simulink model "nms3D_2021"  (R2021a)
settings: Solver=ode15s  StartTime=0.0  StopTime=2  MaxStep=1e-2  RelTol=1e-2
StartFcn:
  | tic
StopFcn:
  | toc
  | 
  | 
  | %if GimbalLockFlag
  |  % fprintf(2, 'Almost reached Gimbal Lock of IMU. Simulation stopped.\n')
  | %end
  | 
  | %fprintf('Elapsed time: %4.2f sec (%4.2f%% realtime)\n', a, tout(end)/a*100)
values from neighbouring files (symbols this model uses):
  Balance02 = pMod(24:29)    [AssignSimulinkParams.m]    (also in assign_parameters.m = param(26:29))
  Balance13 = pMod(30:35)    [AssignSimulinkParams.m]    (also in assign_parameters.m = param(30:33))
  BalanceTrunk = pMod(22:23)    [AssignSimulinkParams.m]    (also in assign_parameters.m = param(22:23))
  BalanceTrunkLat = param(24:25)    [assign_parameters.m]
  BalanceTrunkLatOld = pMod(43:46)    [AssignSimulinkParams.m]    (also in assign_parameters.m = param(43:46))
  BalanceTrunkOld = param(49:53)    [assign_parameters.m]
  BasisStim = pMod(1:11)    [AssignSimulinkParams.m]    (also in assign_parameters.m = param(1:11))
  CompliantLeg = pMod(12:14)    [AssignSimulinkParams.m]    (also in assign_parameters.m = param(12:14))
  CompliantLegLat = pMod(15)    [AssignSimulinkParams.m]    (also in assign_parameters.m = param(15))
  PreventKneeOverextension = pMod(16:21)    [AssignSimulinkParams.m]    (also in assign_parameters.m = param(16:21))
  SwingCompLatOld = param(47:48)    [assign_parameters.m]
  Target02 = pMod(36:38)    [AssignSimulinkParams.m]    (also in assign_parameters.m = param(34:36))
  Target02_va = pMod(49:54)    [AssignSimulinkParams.m]    (also in assign_parameters.m = param(60:65))
  Target13 = pMod(39:41)    [AssignSimulinkParams.m]    (also in assign_parameters.m = param(37:39))
  Target13_va = pMod(55:60)    [AssignSimulinkParams.m]    (also in assign_parameters.m = param(66:71))
  theta0_world = param(59)    [assign_parameters.m]
  WramameiSL_1000 = readmatrix('WSL_1000_Norm_Sigmoid_MSE_cont.csv')    [nms3D_prep.m]
  ZramameiSL_1000 = readmatrix('ZSL_1000_Norm_Sigmoid_MSE_cont.csv')    [nms3D_prep.m]
undefined symbols (not defined in the file or in its folder): ICs, mParams, X, Y, Z
libraries: nesl_utility x106, sm_lib x87, simulink x70, eeGeneralControl x28, robotmaniplib x14, dspinverses x10, robotcorelib x5, dspmathops x3, vrlib x1, pid_lib x1
(part 5 of 8)

== system nms3D_2021/CMA Data/Step Counter/count steps2 ==
  nStep-1 : Inport  LatchByDelayingOutsideSignal=on
  Trigger : TriggerPort  VariantControl=(inherit)  ZeroCross=off
  Constant : Constant
  Sum : Sum  Inputs=|++
  nStep : Outport  InitialOutput=0  VectorParamsAs1DForOutWhenUnconnected=off
  wires:
  Constant/1 -> Sum/2
  nStep-1/1 -> Sum/1
  Sum/1 -> nStep/1

== system nms3D_2021/CMA Data/check steady state/even ==
  In1 : Inport
  Trigger : TriggerPort  TriggerType=falling  VariantControl=(inherit)  ZeroCross=off
  Out1 : Outport  VectorParamsAs1DForOutWhenUnconnected=off
  wires:
  In1/1 -> Out1/1

== system nms3D_2021/CMA Data/check steady state/odd ==
  In1 : Inport
  Trigger : TriggerPort  VariantControl=(inherit)  ZeroCross=off
  Out1 : Outport  VectorParamsAs1DForOutWhenUnconnected=off
  wires:
  In1/1 -> Out1/1

== system nms3D_2021/Muscle Actuation Layer/Muscles Left/Muscle Dynamics (Vectorized)1 ==
  note: Excitation Contraction Coupling
  note: VECTORIZED Muscle-Tendon Dynamics
  lmtc [m] : Inport
  STIM : Inport  Port=2
  1 : Product  Inputs=**  InputSameDT=on  SaturateOnIntegerOverflow=on  OutDataTypeStr=Inherit: Same as first input
  1./lopt : Gain  Gain=1./mParams.muscles.loptVec  SaturateOnIntegerOverflow=on  OutDataTypeStr=Inherit: Same as input  ParamDataTypeStr=Inherit: Same as input
  1./lopt2 : Gain  Gain=1/mParams.muscles.tauA  SaturateOnIntegerOverflow=on  OutDataTypeStr=Inherit: Same as input  ParamDataTypeStr=Inherit: Same as input
  1/lslack : Gain  Gain=1./mParams.muscles.lslackVec  SaturateOnIntegerOverflow=on  OutDataTypeStr=Inherit: Same as input  ParamDataTypeStr=Inherit: Same as input
  BE force-length relation : Subsystem
  CE force-length relation : Subsystem
  CE inverse force-velocity relation : Subsystem
  Constant : Constant  Value=mParams.muscles.lslackVec
  Fmax : Gain  Gain=mParams.muscles.FmaxVec  SaturateOnIntegerOverflow=on  OutDataTypeStr=Inherit: Same as input  ParamDataTypeStr=Inherit: Same as input
  Fv = Fse / (A*Fce) : Product  Inputs=*/  InputSameDT=on  SaturateOnIntegerOverflow=on  OutDataTypeStr=Inherit: Same as first input
  Integrator : Integrator  InitialConditionSource=external  LowerSaturationLimit=0.05
  Integrator1 : Integrator  InitialConditionSource=external  LowerSaturationLimit=0.05
  PE force-length relation : Subsystem
  SE force-length relation : Subsystem
  Sum : Sum  Inputs=|+-  InputSameDT=on  SaturateOnIntegerOverflow=on  OutDataTypeStr=Inherit: Same as first input
  Sum1 : Sum  Inputs=|+-  InputSameDT=on  SaturateOnIntegerOverflow=on  OutDataTypeStr=Inherit: Same as first input
  Sum2 : Sum  Inputs=|-+  InputSameDT=on  SaturateOnIntegerOverflow=on  OutDataTypeStr=Inherit: Same as first input
  Sum3 : Sum  Inputs=+++  InputSameDT=on  SaturateOnIntegerOverflow=on  OutDataTypeStr=Inherit: Same as first input
  Sum4 : Sum  InputSameDT=on  SaturateOnIntegerOverflow=on  OutDataTypeStr=Inherit: Same as first input
  avoid div by 0 : Constant  Value=eps
  preA : Constant  Value=mParams.muscles.preA
  vmax*lopt : Gain  Gain=mParams.muscles.vmaxVec  SaturateOnIntegerOverflow=on  OutDataTypeStr=Inherit: Same as input  ParamDataTypeStr=Inherit: Same as input
  Fmtc : Outport  InitialOutput=0  VectorParamsAs1DForOutWhenUnconnected=off
  Lce : Outport  Port=2  InitialOutput=0  VectorParamsAs1DForOutWhenUnconnected=off
  Vce : Outport  Port=3  InitialOutput=0  VectorParamsAs1DForOutWhenUnconnected=off
  A : Outport  Port=4  InitialOutput=0  VectorParamsAs1DForOutWhenUnconnected=off
  ForceLengthFactor : Outport  Port=5  VectorParamsAs1DForOutWhenUnconnected=off
  tag scope: fl_L=global, fv_L=global
  wires:
  1./lopt2/1 -> Integrator1/1
  Sum1/1 -> 1./lopt2/1
  CE inverse force-velocity relation/1(v[vmax]) -> vmax*lopt/1
  Fv = Fse / (A*Fce)/1 -> CE inverse force-velocity relation/1(Fv[Fmax]), [fv_L]  "fv"
  Sum3/1 -> Fv = Fse / (A*Fce)/2
  Sum4/1 -> Fv = Fse / (A*Fce)/1
  SE force-length relation/1(fse [Fmax]) -> Fmax/1, Sum4/1
  Integrator1/1 -> Sum1/2, A/1, 1/2
  Fmax/1 -> Fmtc/1  "Fmtc"
  lmtc [m]/1 -> Sum/1, Sum2/2  "lmtc"
  vmax*lopt/1 -> Integrator/1, Vce/1  "vce"
  1./lopt/1 -> CE force-length relation/1(lce [lopt]), BE force-length relation/1(lce [lopt]), PE force-length relation/1(lce [lopt])
  Integrator/1 -> 1./lopt/1, Sum/2, Lce/1  "lce"
  1/1 -> Sum3/3
  1/lslack/1 -> SE force-length relation/1(lse [lslack])
  STIM/1 -> Sum1/1
  Sum/1 -> 1/lslack/1  "lse"
  Constant/1 -> Sum2/1
  PE force-length relation/1(fpe [Fmax]) -> Sum3/1
  BE force-length relation/1(fbe [Fmax]) -> Sum4/2
  avoid div by 0/1 -> Sum3/2
  preA/1 -> Integrator1/2
  Sum2/1 -> Integrator/2
  CE force-length relation/1(fce [Fmax]) -> [fl_L], ForceLengthFactor/1, 1/1

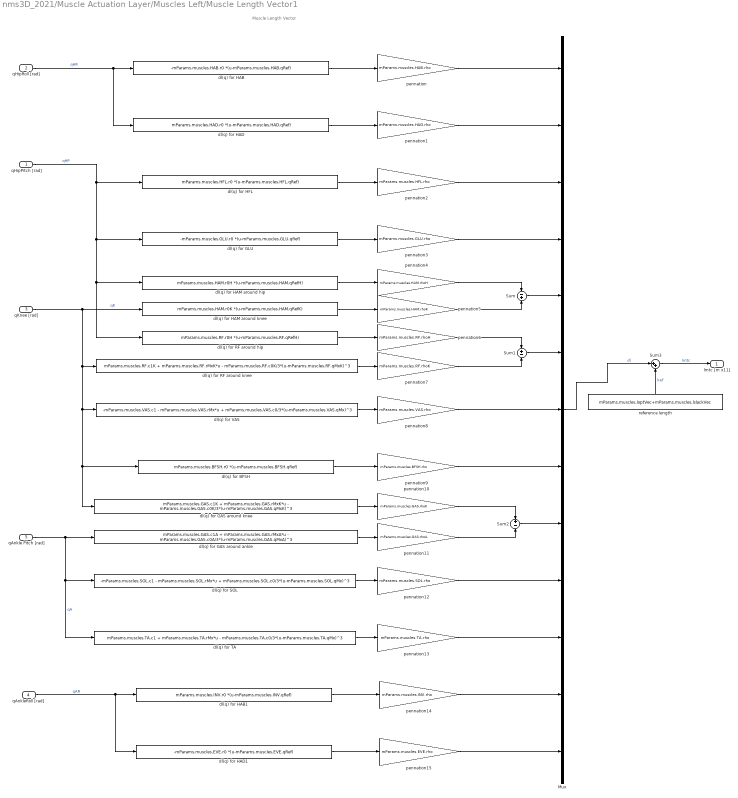
== system nms3D_2021/Muscle Actuation Layer/Muscles Left/Muscle Length Vector1 ==
  note: Muscle Length Vector
  qHipPitch [rad] : Inport
  qHipRoll [rad] : Inport  Port=2
  qKnee [rad] : Inport  Port=3
  qAnkleRoll [rad] : Inport  Port=4
  qAnkle Pitch [rad] : Inport  Port=5
  Mux : Mux  Inputs=13
  Sum : Sum  Inputs=-+
  Sum1 : Sum  Inputs=+-
  Sum2 : Sum  Inputs=+-
  Sum3 : Sum  Inputs=|++
  dl(q) for BFSH : Fcn  Expr=mParams.muscles.BFSH.r0 *(u-mParams.muscles.BFSH.qRef)
  dl(q) for GAS around ankle : Fcn  Expr=mParams.muscles.GAS.c1A + mParams.muscles.GAS.rMxA*u - mParams.muscles.GAS.c0A/3*(u-mParams.muscles.GAS.qMxA)^3
  dl(q) for GAS around knee : Fcn  Expr=mParams.muscles.GAS.c1K + mParams.muscles.GAS.rMxK*u - mParams.muscles.GAS.c0K/3*(u-mParams.muscles.GAS.qMxK)^3
  dl(q) for GLU : Fcn  Expr=-mParams.muscles.GLU.r0 *(u-mParams.muscles.GLU.qRef)
  dl(q) for HAB : Fcn  Expr=-mParams.muscles.HAB.r0 *(u-mParams.muscles.HAB.qRef)
  dl(q) for HAB1 : Fcn  Expr=mParams.muscles.INV.r0 *(u-mParams.muscles.INV.qRef)
  dl(q) for HAD : Fcn  Expr=mParams.muscles.HAD.r0 *(u-mParams.muscles.HAD.qRef)
  dl(q) for HAD1 : Fcn  Expr=-mParams.muscles.EVE.r0 *(u-mParams.muscles.EVE.qRef)
  dl(q) for HAM around hip : Fcn  Expr=mParams.muscles.HAM.r0H *(u-mParams.muscles.HAM.qRefH)
  dl(q) for HAM around knee : Fcn  Expr=mParams.muscles.HAM.r0K *(u-mParams.muscles.HAM.qRefK)
  dl(q) for HFL : Fcn  Expr=mParams.muscles.HFL.r0 *(u-mParams.muscles.HFL.qRef)
  dl(q) for RF around hip : Fcn  Expr=mParams.muscles.RF.r0H *(u-mParams.muscles.RF.qRefH)
  dl(q) for RF around knee : Fcn  Expr=mParams.muscles.RF.c1K + mParams.muscles.RF.rMxK*u - mParams.muscles.RF.c0K/3*(u-mParams.muscles.RF.qMxK)^3
  dl(q) for SOL : Fcn  Expr=-mParams.muscles.SOL.c1 - mParams.muscles.SOL.rMx*u + mParams.muscles.SOL.c0/3*(u-mParams.muscles.SOL.qMx)^3
  dl(q) for TA : Fcn  Expr=mParams.muscles.TA.c1 + mParams.muscles.TA.rMx*u - mParams.muscles.TA.c0/3*(u-mParams.muscles.TA.qMx)^3
  dl(q) for VAS : Fcn  Expr=-mParams.muscles.VAS.c1 - mParams.muscles.VAS.rMx*u + mParams.muscles.VAS.c0/3*(u-mParams.muscles.VAS.qMx)^3
  pennation : Gain  Gain=mParams.muscles.HAB.rho
  pennation1 : Gain  Gain=mParams.muscles.HAD.rho
  pennation10 : Gain  Gain=mParams.muscles.GAS.rhoK
  pennation11 : Gain  Gain=mParams.muscles.GAS.rhoA
  pennation12 : Gain  Gain=mParams.muscles.SOL.rho
  pennation13 : Gain  Gain=mParams.muscles.TA.rho
  pennation14 : Gain  Gain=mParams.muscles.INV.rho
  pennation15 : Gain  Gain=mParams.muscles.EVE.rho
  pennation2 : Gain  Gain=mParams.muscles.HFL.rho
  pennation3 : Gain  Gain=mParams.muscles.GLU.rho
  pennation4 : Gain  Gain=mParams.muscles.HAM.rhoH
  pennation5 : Gain  Gain=mParams.muscles.HAM.rhoK
  pennation6 : Gain  Gain=mParams.muscles.RF.rhoH
  pennation7 : Gain  Gain=mParams.muscles.RF.rhoK
  pennation8 : Gain  Gain=mParams.muscles.VAS.rho
  pennation9 : Gain  Gain=mParams.muscles.BFSH.rho
  reference length : Constant  Value=mParams.muscles.loptVec+mParams.muscles.lslackVec
  lmtc [m x11] : Outport  VectorParamsAs1DForOutWhenUnconnected=off
  wires:
  dl(q) for HAB/1 -> pennation/1
  dl(q) for HFL/1 -> pennation2/1
  dl(q) for HAM around knee/1 -> pennation5/1
  dl(q) for BFSH/1 -> pennation9/1
  dl(q) for HAM around hip/1 -> pennation4/1
  qAnkle Pitch [rad]/1 -> dl(q) for TA/1, dl(q) for SOL/1, dl(q) for GAS around ankle/1  "qA"
  dl(q) for TA/1 -> pennation13/1
  dl(q) for HAD/1 -> pennation1/1
  dl(q) for GLU/1 -> pennation3/1
  dl(q) for RF around knee/1 -> pennation7/1
  dl(q) for SOL/1 -> pennation12/1
  qHipPitch [rad]/1 -> dl(q) for RF around hip/1, dl(q) for HAM around hip/1, dl(q) for GLU/1, dl(q) for HFL/1  "qHP"
  dl(q) for RF around hip/1 -> pennation6/1
  qHipRoll [rad]/1 -> dl(q) for HAD/1, dl(q) for HAB/1  "qHR"
  Sum1/1 -> Mux/6
  qKnee [rad]/1 -> dl(q) for GAS around knee/1, dl(q) for BFSH/1, dl(q) for VAS/1, dl(q) for RF around knee/1, dl(q) for HAM around knee/1  "qK"
  Sum/1 -> Mux/5
  Sum2/1 -> Mux/9
  dl(q) for GAS around knee/1 -> pennation10/1
  dl(q) for GAS around ankle/1 -> pennation11/1
  dl(q) for VAS/1 -> pennation8/1
  Mux/1 -> Sum3/1  "dl"
  Sum3/1 -> lmtc [m x11]/1  "lmtc"
  reference length/1 -> Sum3/2  "lref"
  pennation/1 -> Mux/1
  pennation1/1 -> Mux/2
  pennation2/1 -> Mux/3
  pennation3/1 -> Mux/4
  pennation4/1 -> Sum/1
  pennation5/1 -> Sum/2
  pennation6/1 -> Sum1/1
  pennation7/1 -> Sum1/2
  pennation8/1 -> Mux/7
  pennation9/1 -> Mux/8
  pennation10/1 -> Sum2/1
  pennation11/1 -> Sum2/2
  pennation12/1 -> Mux/10
  pennation13/1 -> Mux/11
  qAnkleRoll [rad]/1 -> dl(q) for HAD1/1, dl(q) for HAB1/1  "qAR"
  pennation15/1 -> Mux/13
  dl(q) for HAB1/1 -> pennation14/1
  dl(q) for HAD1/1 -> pennation15/1
  pennation14/1 -> Mux/12

== system nms3D_2021/Muscle Actuation Layer/Muscles Left/Muscle Torque Contributions1 ==
  note: Leg Muscle Torque Contributions
  qKnee [rad] : Inport
  qAnkle [rad] : Inport  Port=2
  FmVec [N x11] : Inport  Port=3
  Demux1 : Demux  Outputs=13
  Product{1..6} (6 alike) : Product
  Subsystem : Subsystem
  Sum : Sum  Inputs=+-
  Sum1 : Sum  Inputs=-++-
  Sum2 : Sum  Inputs=-++--
  Sum3 : Sum  Inputs=++-
  Sum4 : Sum  Inputs=-+
  r(q) RF around knee : Fcn  Expr=mParams.muscles.RF.rMxK - mParams.muscles.RF.c0K*(u-mParams.muscles.RF.qMxK)^2
  r(q) RGAS around ankle : Fcn  Expr=mParams.muscles.GAS.rMxA - mParams.muscles.GAS.c0A*(u-mParams.muscles.GAS.qMxA)^2
  r(q) RGAS around knee : Fcn  Expr=mParams.muscles.GAS.rMxK - mParams.muscles.GAS.c0K*(u-mParams.muscles.GAS.qMxK)^2
  r(q) RSOL : Fcn  Expr=mParams.muscles.SOL.rMx - mParams.muscles.SOL.c0*(u-mParams.muscles.SOL.qMx)^2
  r(q) RTA : Fcn  Expr=mParams.muscles.TA.rMx - mParams.muscles.TA.c0*(u-mParams.muscles.TA.qMx)^2
  r(q) for BFSH : Gain  Gain=mParams.muscles.BFSH.r0
  r(q) for EVE : Gain  Gain=mParams.muscles.INV.r0
  r(q) for GLU : Gain  Gain=mParams.muscles.GLU.r0
  r(q) for HAB : Gain  Gain=mParams.muscles.HAB.r0
  r(q) for HAD : Gain  Gain=mParams.muscles.HAD.r0
  r(q) for HAD1 : Gain  Gain=mParams.muscles.EVE.r0
  r(q) for HAM at hip : Gain  Gain=mParams.muscles.HAM.r0H
  r(q) for HAM at knee : Gain  Gain=mParams.muscles.HAM.r0K
  r(q) for HFL : Gain  Gain=mParams.muscles.HFL.r0
  r(q) for RF : Gain  Gain=mParams.muscles.RF.r0H
  r(q) for VAS : Fcn  Expr=mParams.muscles.VAS.rMx - mParams.muscles.VAS.c0*(u-mParams.muscles.VAS.qMx)^2
  tauHP [Nm] : Outport  VectorParamsAs1DForOutWhenUnconnected=off
  tauHR [Nm] : Outport  Port=2  VectorParamsAs1DForOutWhenUnconnected=off
  tauK [Nm] : Outport  Port=3  VectorParamsAs1DForOutWhenUnconnected=off
  tauAR [Nm] : Outport  Port=4  VectorParamsAs1DForOutWhenUnconnected=off
  tauA [Nm] : Outport  Port=5  VectorParamsAs1DForOutWhenUnconnected=off
  Leg Torque : Outport  Port=6  VectorParamsAs1DForOutWhenUnconnected=off
  wires:
  qKnee [rad]/1 -> r(q) RGAS around knee/1, r(q) RF around knee/1, r(q) for VAS/1  "qK"
  qAnkle [rad]/1 -> r(q) RTA/1, r(q) RSOL/1, r(q) RGAS around ankle/1  "qA"
  FmVec [N x11]/1 -> Demux1/1
  Demux1/1 -> r(q) for HAB/1  "HAB"
  Demux1/2 -> r(q) for HAD/1  "HAD"
  r(q) for HAD/1 -> Sum/2
  r(q) for HAB/1 -> Sum/1
  Demux1/3 -> r(q) for HFL/1  "HFL"
  Demux1/4 -> r(q) for GLU/1  "GLU"
  Demux1/5 -> r(q) for HAM at knee/1, r(q) for HAM at hip/1  "HAM"
  Demux1/6 -> Product1/1, r(q) for RF/1  "RF"
  r(q) for RF/1 -> Sum1/4
  r(q) RF around knee/1 -> Product1/2
  Product1/1 -> Sum2/2
  r(q) for HAM at knee/1 -> Sum2/1
  r(q) for HAM at hip/1 -> Sum1/3
  r(q) for GLU/1 -> Sum1/2
  r(q) for HFL/1 -> Sum1/1
  Sum1/1 -> tauHP [Nm]/1
  Demux1/7 -> Subsystem/1(F VAS), Product2/1  "VAS"
  r(q) for VAS/1 -> Subsystem/2(Moment Arm VAS), Product2/2
  Demux1/8 -> r(q) for BFSH/1  "BFSH"
  Demux1/9 -> Product3/1, Product4/1  "GAS"
  r(q) RGAS around knee/1 -> Product3/2
  Product2/1 -> Sum2/3
  r(q) for BFSH/1 -> Sum2/4
  Product3/1 -> Sum2/5
  Sum2/1 -> tauK [Nm]/1
  r(q) RGAS around ankle/1 -> Product4/2
  r(q) RSOL/1 -> Product5/2, Subsystem/4(Moment Arm SOL)
  Demux1/10 -> Subsystem/3(F SOL), Product5/1  "SOL"
  r(q) RTA/1 -> Product6/2
  Demux1/11 -> Product6/1  "TA"
  Product4/1 -> Sum3/1
  Product5/1 -> Sum3/2
  Product6/1 -> Sum3/3
  Sum3/1 -> tauA [Nm]/1
  Sum/1 -> tauHR [Nm]/1
  Subsystem/1("Leg Torque ") -> Leg Torque/1
  Demux1/13 -> r(q) for HAD1/1  "EVE"
  Sum4/1 -> tauAR [Nm]/1
  r(q) for HAD1/1 -> Sum4/2
  r(q) for EVE/1 -> Sum4/1
  Demux1/12 -> r(q) for EVE/1  "INV"

== system nms3D_2021/Muscle Actuation Layer/Muscles Right/Muscle Dynamics (Vectorized) ==
  note: Excitation Contraction Coupling
  lmtc [m] : Inport
  STIM : Inport  Port=2
  1 : Product  Inputs=**  InputSameDT=on  SaturateOnIntegerOverflow=on  OutDataTypeStr=Inherit: Same as first input
  1./lopt : Gain  Gain=1./mParams.muscles.loptVec  SaturateOnIntegerOverflow=on  OutDataTypeStr=Inherit: Same as input  ParamDataTypeStr=Inherit: Same as input
  1./lopt2 : Gain  Gain=1/mParams.muscles.tauA  SaturateOnIntegerOverflow=on  OutDataTypeStr=Inherit: Same as input  ParamDataTypeStr=Inherit: Same as input
  1/lslack : Gain  Gain=1./mParams.muscles.lslackVec  SaturateOnIntegerOverflow=on  OutDataTypeStr=Inherit: Same as input  ParamDataTypeStr=Inherit: Same as input
  BE force-length relation : Subsystem
  CE force-length relation : Subsystem
  CE inverse force-velocity relation : Subsystem
  Constant : Constant  Value=mParams.muscles.lslackVec
  Fmax : Gain  Gain=mParams.muscles.FmaxVec  SaturateOnIntegerOverflow=on  OutDataTypeStr=Inherit: Same as input  ParamDataTypeStr=Inherit: Same as input
  Fv = Fse / (A*Fce) : Product  Inputs=*/  InputSameDT=on  SaturateOnIntegerOverflow=on  OutDataTypeStr=Inherit: Same as first input
  Integrator : Integrator  InitialConditionSource=external  LowerSaturationLimit=0.05
  Integrator1 : Integrator  InitialConditionSource=external  LowerSaturationLimit=0.05
  PE force-length relation : Subsystem
  SE force-length relation : Subsystem
  Sum : Sum  Inputs=|+-  InputSameDT=on  SaturateOnIntegerOverflow=on  OutDataTypeStr=Inherit: Same as first input
  Sum1 : Sum  Inputs=|+-  InputSameDT=on  SaturateOnIntegerOverflow=on  OutDataTypeStr=Inherit: Same as first input
  Sum2 : Sum  Inputs=|-+  InputSameDT=on  SaturateOnIntegerOverflow=on  OutDataTypeStr=Inherit: Same as first input
  Sum3 : Sum  Inputs=+++  InputSameDT=on  SaturateOnIntegerOverflow=on  OutDataTypeStr=Inherit: Same as first input
  Sum4 : Sum  InputSameDT=on  SaturateOnIntegerOverflow=on  OutDataTypeStr=Inherit: Same as first input
  avoid div by 0 : Constant  Value=eps
  preA : Constant  Value=mParams.muscles.preA
  vmax*lopt : Gain  Gain=mParams.muscles.vmaxVec  SaturateOnIntegerOverflow=on  OutDataTypeStr=Inherit: Same as input  ParamDataTypeStr=Inherit: Same as input
  Fmtc : Outport  InitialOutput=0  VectorParamsAs1DForOutWhenUnconnected=off
  Lce : Outport  Port=2  InitialOutput=0  VectorParamsAs1DForOutWhenUnconnected=off
  Vce : Outport  Port=3  InitialOutput=0  VectorParamsAs1DForOutWhenUnconnected=off
  A : Outport  Port=4  InitialOutput=0  VectorParamsAs1DForOutWhenUnconnected=off
  ForceLengthFactor : Outport  Port=5  VectorParamsAs1DForOutWhenUnconnected=off
  tag scope: fl_R=global, fv_R=global
  wires:
  1./lopt2/1 -> Integrator1/1
  Sum1/1 -> 1./lopt2/1
  CE inverse force-velocity relation/1(v[vmax]) -> vmax*lopt/1
  Fv = Fse / (A*Fce)/1 -> CE inverse force-velocity relation/1(Fv[Fmax]), [fv_R]  "fv"
  Sum3/1 -> Fv = Fse / (A*Fce)/2
  Sum4/1 -> Fv = Fse / (A*Fce)/1
  SE force-length relation/1(fse [Fmax]) -> Fmax/1, Sum4/1
  STIM/1 -> Sum1/1
  Integrator1/1 -> Sum1/2, A/1, 1/2
  1/lslack/1 -> SE force-length relation/1(lse [lslack])
  Fmax/1 -> Fmtc/1  "Fmtc"
  lmtc [m]/1 -> Sum2/2, Sum/1  "lmtc"
  vmax*lopt/1 -> Vce/1, Integrator/1  "vce"
  1./lopt/1 -> CE force-length relation/1(lce [lopt]), PE force-length relation/1(lce [lopt]), BE force-length relation/1(lce [lopt])
  Integrator/1 -> Lce/1, 1./lopt/1, Sum/2  "lce"
  1/1 -> Sum3/3
  avoid div by 0/1 -> Sum3/2
  Sum2/1 -> Integrator/2
  Sum/1 -> 1/lslack/1  "lse"
  Constant/1 -> Sum2/1
  PE force-length relation/1(fpe [Fmax]) -> Sum3/1
  BE force-length relation/1(fbe [Fmax]) -> Sum4/2
  preA/1 -> Integrator1/2
  CE force-length relation/1(fce [Fmax]) -> [fl_R], ForceLengthFactor/1, 1/1

== system nms3D_2021/Muscle Actuation Layer/Muscles Right/Muscle Length Vector ==
  note: Muscle Length Vector
  note: Muscle Length Vector
  qHipPitch [rad] : Inport
  qHipRoll [rad] : Inport  Port=2
  qKnee [rad] : Inport  Port=3
  qAnkle [rad] : Inport  Port=4
  Mux : Mux  Inputs=11
  Sum : Sum  Inputs=-+
  Sum1 : Sum  Inputs=+-
  Sum2 : Sum  Inputs=+-
  Sum3 : Sum  Inputs=|++
  dl(q) for BFSH : Fcn  Expr=mParams.muscles.BFSH.r0 *(u-mParams.muscles.BFSH.qRef)
  dl(q) for GAS around ankle : Fcn  Expr=mParams.muscles.GAS.c1A + mParams.muscles.GAS.rMxA*u - mParams.muscles.GAS.c0A/3*(u-mParams.muscles.GAS.qMxA)^3
  dl(q) for GAS around knee : Fcn  Expr=mParams.muscles.GAS.c1K + mParams.muscles.GAS.rMxK*u - mParams.muscles.GAS.c0K/3*(u-mParams.muscles.GAS.qMxK)^3
  dl(q) for GLU : Fcn  Expr=-mParams.muscles.GLU.r0 *(u-mParams.muscles.GLU.qRef)
  dl(q) for HAB : Fcn  Expr=-mParams.muscles.HAB.r0 *(u-mParams.muscles.HAB.qRef)
  dl(q) for HAD : Fcn  Expr=mParams.muscles.HAD.r0 *(u-mParams.muscles.HAD.qRef)
  dl(q) for HAM around hip : Fcn  Expr=mParams.muscles.HAM.r0H *(u-mParams.muscles.HAM.qRefH)
  dl(q) for HAM around knee : Fcn  Expr=mParams.muscles.HAM.r0K *(u-mParams.muscles.HAM.qRefK)
  dl(q) for HFL : Fcn  Expr=mParams.muscles.HFL.r0 *(u-mParams.muscles.HFL.qRef)
  dl(q) for RF around hip : Fcn  Expr=mParams.muscles.RF.r0H *(u-mParams.muscles.RF.qRefH)
  dl(q) for RF around knee : Fcn  Expr=mParams.muscles.RF.c1K + mParams.muscles.RF.rMxK*u - mParams.muscles.RF.c0K/3*(u-mParams.muscles.RF.qMxK)^3
  dl(q) for SOL : Fcn  Expr=-mParams.muscles.SOL.c1 - mParams.muscles.SOL.rMx*u + mParams.muscles.SOL.c0/3*(u-mParams.muscles.SOL.qMx)^3
  dl(q) for TA : Fcn  Expr=mParams.muscles.TA.c1 + mParams.muscles.TA.rMx*u - mParams.muscles.TA.c0/3*(u-mParams.muscles.TA.qMx)^3
  dl(q) for VAS : Fcn  Expr=-mParams.muscles.VAS.c1 - mParams.muscles.VAS.rMx*u + mParams.muscles.VAS.c0/3*(u-mParams.muscles.VAS.qMx)^3
  pennation : Gain  Gain=mParams.muscles.HAB.rho
  pennation1 : Gain  Gain=mParams.muscles.HAD.rho
  pennation10 : Gain  Gain=mParams.muscles.GAS.rhoK
  pennation11 : Gain  Gain=mParams.muscles.GAS.rhoA
  pennation12 : Gain  Gain=mParams.muscles.SOL.rho
  pennation13 : Gain  Gain=mParams.muscles.TA.rho
  pennation2 : Gain  Gain=mParams.muscles.HFL.rho
  pennation3 : Gain  Gain=mParams.muscles.GLU.rho
  pennation4 : Gain  Gain=mParams.muscles.HAM.rhoH
  pennation5 : Gain  Gain=mParams.muscles.HAM.rhoK
  pennation6 : Gain  Gain=mParams.muscles.RF.rhoH
  pennation7 : Gain  Gain=mParams.muscles.RF.rhoK
  pennation8 : Gain  Gain=mParams.muscles.VAS.rho
  pennation9 : Gain  Gain=mParams.muscles.BFSH.rho
  reference length : Constant  Value=mParams.muscles.loptVec+mParams.muscles.lslackVec
  lmtc [m x11] : Outport  VectorParamsAs1DForOutWhenUnconnected=off
  wires:
  dl(q) for HAB/1 -> pennation/1
  dl(q) for HFL/1 -> pennation2/1
  dl(q) for HAM around knee/1 -> pennation5/1
  dl(q) for BFSH/1 -> pennation9/1
  dl(q) for HAM around hip/1 -> pennation4/1
  qAnkle [rad]/1 -> dl(q) for TA/1, dl(q) for SOL/1, dl(q) for GAS around ankle/1  "qA"
  dl(q) for TA/1 -> pennation13/1
  dl(q) for HAD/1 -> pennation1/1
  dl(q) for GLU/1 -> pennation3/1
  dl(q) for RF around knee/1 -> pennation7/1
  dl(q) for SOL/1 -> pennation12/1
  qHipPitch [rad]/1 -> dl(q) for HAM around hip/1, dl(q) for RF around hip/1, dl(q) for GLU/1, dl(q) for HFL/1  "qHP"
  dl(q) for RF around hip/1 -> pennation6/1
  qHipRoll [rad]/1 -> dl(q) for HAD/1, dl(q) for HAB/1  "qHR"
  Sum1/1 -> Mux/6
  qKnee [rad]/1 -> dl(q) for HAM around knee/1, dl(q) for VAS/1, dl(q) for GAS around knee/1, dl(q) for BFSH/1, dl(q) for RF around knee/1  "qK"
  Sum/1 -> Mux/5
  Sum2/1 -> Mux/9
  dl(q) for GAS around knee/1 -> pennation10/1
  dl(q) for GAS around ankle/1 -> pennation11/1
  dl(q) for VAS/1 -> pennation8/1
  Mux/1 -> Sum3/1  "dl"
  Sum3/1 -> lmtc [m x11]/1  "lmtc"
  reference length/1 -> Sum3/2  "lref"
  pennation2/1 -> Mux/3
  pennation3/1 -> Mux/4
  pennation4/1 -> Sum/1
  pennation5/1 -> Sum/2
  pennation6/1 -> Sum1/1
  pennation7/1 -> Sum1/2
  pennation8/1 -> Mux/7
  pennation9/1 -> Mux/8
  pennation10/1 -> Sum2/1
  pennation11/1 -> Sum2/2
  pennation12/1 -> Mux/10
  pennation13/1 -> Mux/11
  pennation/1 -> Mux/1
  pennation1/1 -> Mux/2

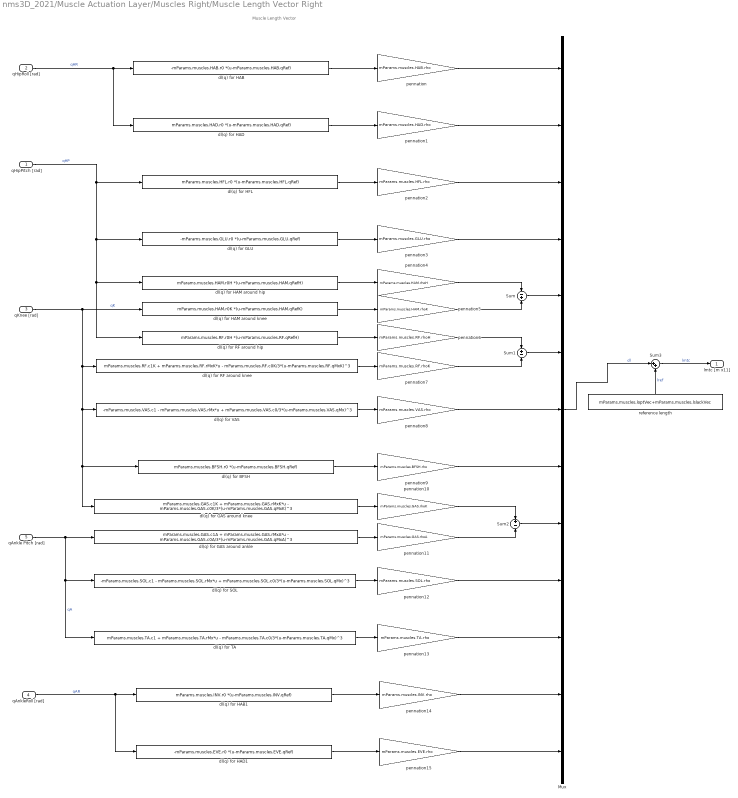
== system nms3D_2021/Muscle Actuation Layer/Muscles Right/Muscle Length Vector Right ==
  note: Muscle Length Vector
  qHipPitch [rad] : Inport
  qHipRoll [rad] : Inport  Port=2
  qKnee [rad] : Inport  Port=3
  qAnkleRoll [rad] : Inport  Port=4
  qAnkle Pitch [rad] : Inport  Port=5
  Mux : Mux  Inputs=13
  Sum : Sum  Inputs=-+
  Sum1 : Sum  Inputs=+-
  Sum2 : Sum  Inputs=+-
  Sum3 : Sum  Inputs=|++
  dl(q) for BFSH : Fcn  Expr=mParams.muscles.BFSH.r0 *(u-mParams.muscles.BFSH.qRef)
  dl(q) for GAS around ankle : Fcn  Expr=mParams.muscles.GAS.c1A + mParams.muscles.GAS.rMxA*u - mParams.muscles.GAS.c0A/3*(u-mParams.muscles.GAS.qMxA)^3
  dl(q) for GAS around knee : Fcn  Expr=mParams.muscles.GAS.c1K + mParams.muscles.GAS.rMxK*u - mParams.muscles.GAS.c0K/3*(u-mParams.muscles.GAS.qMxK)^3
  dl(q) for GLU : Fcn  Expr=-mParams.muscles.GLU.r0 *(u-mParams.muscles.GLU.qRef)
  dl(q) for HAB : Fcn  Expr=-mParams.muscles.HAB.r0 *(u-mParams.muscles.HAB.qRef)
  dl(q) for HAB1 : Fcn  Expr=mParams.muscles.INV.r0 *(u-mParams.muscles.INV.qRef)
  dl(q) for HAD : Fcn  Expr=mParams.muscles.HAD.r0 *(u-mParams.muscles.HAD.qRef)
  dl(q) for HAD1 : Fcn  Expr=-mParams.muscles.EVE.r0 *(u-mParams.muscles.EVE.qRef)
  dl(q) for HAM around hip : Fcn  Expr=mParams.muscles.HAM.r0H *(u-mParams.muscles.HAM.qRefH)
  dl(q) for HAM around knee : Fcn  Expr=mParams.muscles.HAM.r0K *(u-mParams.muscles.HAM.qRefK)
  dl(q) for HFL : Fcn  Expr=mParams.muscles.HFL.r0 *(u-mParams.muscles.HFL.qRef)
  dl(q) for RF around hip : Fcn  Expr=mParams.muscles.RF.r0H *(u-mParams.muscles.RF.qRefH)
  dl(q) for RF around knee : Fcn  Expr=mParams.muscles.RF.c1K + mParams.muscles.RF.rMxK*u - mParams.muscles.RF.c0K/3*(u-mParams.muscles.RF.qMxK)^3
  dl(q) for SOL : Fcn  Expr=-mParams.muscles.SOL.c1 - mParams.muscles.SOL.rMx*u + mParams.muscles.SOL.c0/3*(u-mParams.muscles.SOL.qMx)^3
  dl(q) for TA : Fcn  Expr=mParams.muscles.TA.c1 + mParams.muscles.TA.rMx*u - mParams.muscles.TA.c0/3*(u-mParams.muscles.TA.qMx)^3
  dl(q) for VAS : Fcn  Expr=-mParams.muscles.VAS.c1 - mParams.muscles.VAS.rMx*u + mParams.muscles.VAS.c0/3*(u-mParams.muscles.VAS.qMx)^3
  pennation : Gain  Gain=mParams.muscles.HAB.rho
  pennation1 : Gain  Gain=mParams.muscles.HAD.rho
  pennation10 : Gain  Gain=mParams.muscles.GAS.rhoK
  pennation11 : Gain  Gain=mParams.muscles.GAS.rhoA
  pennation12 : Gain  Gain=mParams.muscles.SOL.rho
  pennation13 : Gain  Gain=mParams.muscles.TA.rho
  pennation14 : Gain  Gain=mParams.muscles.INV.rho
  pennation15 : Gain  Gain=mParams.muscles.EVE.rho
  pennation2 : Gain  Gain=mParams.muscles.HFL.rho
  pennation3 : Gain  Gain=mParams.muscles.GLU.rho
  pennation4 : Gain  Gain=mParams.muscles.HAM.rhoH
  pennation5 : Gain  Gain=mParams.muscles.HAM.rhoK
  pennation6 : Gain  Gain=mParams.muscles.RF.rhoH
  pennation7 : Gain  Gain=mParams.muscles.RF.rhoK
  pennation8 : Gain  Gain=mParams.muscles.VAS.rho
  pennation9 : Gain  Gain=mParams.muscles.BFSH.rho
  reference length : Constant  Value=mParams.muscles.loptVec+mParams.muscles.lslackVec
  lmtc [m x11] : Outport  VectorParamsAs1DForOutWhenUnconnected=off
  wires:
  dl(q) for HAB/1 -> pennation/1
  dl(q) for HFL/1 -> pennation2/1
  dl(q) for HAM around knee/1 -> pennation5/1
  dl(q) for BFSH/1 -> pennation9/1
  dl(q) for HAM around hip/1 -> pennation4/1
  qAnkle Pitch [rad]/1 -> dl(q) for TA/1, dl(q) for SOL/1, dl(q) for GAS around ankle/1  "qA"
  dl(q) for TA/1 -> pennation13/1
  dl(q) for HAD/1 -> pennation1/1
  dl(q) for GLU/1 -> pennation3/1
  dl(q) for RF around knee/1 -> pennation7/1
  dl(q) for SOL/1 -> pennation12/1
  qHipPitch [rad]/1 -> dl(q) for RF around hip/1, dl(q) for HAM around hip/1, dl(q) for GLU/1, dl(q) for HFL/1  "qHP"
  dl(q) for RF around hip/1 -> pennation6/1
  qHipRoll [rad]/1 -> dl(q) for HAD/1, dl(q) for HAB/1  "qHR"
  Sum1/1 -> Mux/6
  qKnee [rad]/1 -> dl(q) for GAS around knee/1, dl(q) for BFSH/1, dl(q) for VAS/1, dl(q) for RF around knee/1, dl(q) for HAM around knee/1  "qK"
  Sum/1 -> Mux/5
  Sum2/1 -> Mux/9
  dl(q) for GAS around knee/1 -> pennation10/1
  dl(q) for GAS around ankle/1 -> pennation11/1
  dl(q) for VAS/1 -> pennation8/1
  Mux/1 -> Sum3/1  "dl"
  Sum3/1 -> lmtc [m x11]/1  "lmtc"
  reference length/1 -> Sum3/2  "lref"
  pennation/1 -> Mux/1
  pennation1/1 -> Mux/2
  pennation2/1 -> Mux/3
  pennation3/1 -> Mux/4
  pennation4/1 -> Sum/1
  pennation5/1 -> Sum/2
  pennation6/1 -> Sum1/1
  pennation7/1 -> Sum1/2
  pennation8/1 -> Mux/7
  pennation9/1 -> Mux/8
  pennation10/1 -> Sum2/1
  pennation11/1 -> Sum2/2
  pennation12/1 -> Mux/10
  pennation13/1 -> Mux/11
  qAnkleRoll [rad]/1 -> dl(q) for HAD1/1, dl(q) for HAB1/1  "qAR"
  pennation15/1 -> Mux/13
  dl(q) for HAB1/1 -> pennation14/1
  dl(q) for HAD1/1 -> pennation15/1
  pennation14/1 -> Mux/12

== system nms3D_2021/Muscle Actuation Layer/Muscles Right/Muscle Torque Contributions ==
  note: Leg Muscle Torque Contributions
  qKnee [rad] : Inport
  qAnkle [rad] : Inport  Port=2
  FmVec [N x11] : Inport  Port=3
  Demux1 : Demux  Outputs=13
  Product{1..6} (6 alike) : Product
  Subsystem : Subsystem
  Sum : Sum  Inputs=+-
  Sum1 : Sum  Inputs=-++-
  Sum2 : Sum  Inputs=-++--
  Sum3 : Sum  Inputs=++-
  Sum4 : Sum  Inputs=-+
  r(q) RF around knee : Fcn  Expr=mParams.muscles.RF.rMxK - mParams.muscles.RF.c0K*(u-mParams.muscles.RF.qMxK)^2
  r(q) RGAS around ankle : Fcn  Expr=mParams.muscles.GAS.rMxA - mParams.muscles.GAS.c0A*(u-mParams.muscles.GAS.qMxA)^2
  r(q) RGAS around knee : Fcn  Expr=mParams.muscles.GAS.rMxK - mParams.muscles.GAS.c0K*(u-mParams.muscles.GAS.qMxK)^2
  r(q) RSOL : Fcn  Expr=mParams.muscles.SOL.rMx - mParams.muscles.SOL.c0*(u-mParams.muscles.SOL.qMx)^2
  r(q) RTA : Fcn  Expr=mParams.muscles.TA.rMx - mParams.muscles.TA.c0*(u-mParams.muscles.TA.qMx)^2
  r(q) for BFSH : Gain  Gain=mParams.muscles.BFSH.r0
  r(q) for GLU : Gain  Gain=mParams.muscles.GLU.r0
  r(q) for HAB : Gain  Gain=mParams.muscles.HAB.r0
  r(q) for HAB1 : Gain  Gain=mParams.muscles.INV.r0
  r(q) for HAD : Gain  Gain=mParams.muscles.HAD.r0
  r(q) for HAD1 : Gain  Gain=mParams.muscles.EVE.r0
  r(q) for HAM at hip : Gain  Gain=mParams.muscles.HAM.r0H
  r(q) for HAM at knee : Gain  Gain=mParams.muscles.HAM.r0K
  r(q) for HFL : Gain  Gain=mParams.muscles.HFL.r0
  r(q) for RF : Gain  Gain=mParams.muscles.RF.r0H
  r(q) for VAS : Fcn  Expr=mParams.muscles.VAS.rMx - mParams.muscles.VAS.c0*(u-mParams.muscles.VAS.qMx)^2
  tauHP [Nm] : Outport  VectorParamsAs1DForOutWhenUnconnected=off
  tauHR [Nm] : Outport  Port=2  VectorParamsAs1DForOutWhenUnconnected=off
  tauK [Nm] : Outport  Port=3  VectorParamsAs1DForOutWhenUnconnected=off
  tauAR [Nm] : Outport  Port=4  VectorParamsAs1DForOutWhenUnconnected=off
  tauA [Nm] : Outport  Port=5  VectorParamsAs1DForOutWhenUnconnected=off
  Leg Torque : Outport  Port=6  VectorParamsAs1DForOutWhenUnconnected=off
  wires:
  qKnee [rad]/1 -> r(q) RGAS around knee/1, r(q) RF around knee/1, r(q) for VAS/1  "qK"
  qAnkle [rad]/1 -> r(q) RTA/1, r(q) RSOL/1, r(q) RGAS around ankle/1  "qA"
  FmVec [N x11]/1 -> Demux1/1
  Demux1/1 -> r(q) for HAB/1  "HAB"
  Demux1/2 -> r(q) for HAD/1  "HAD"
  r(q) for HAD/1 -> Sum/2
  r(q) for HAB/1 -> Sum/1
  Demux1/3 -> r(q) for HFL/1  "HFL"
  Demux1/4 -> r(q) for GLU/1  "GLU"
  Demux1/5 -> r(q) for HAM at knee/1, r(q) for HAM at hip/1  "HAM"
  Demux1/6 -> Product1/1, r(q) for RF/1  "RF"
  r(q) for RF/1 -> Sum1/4
  r(q) RF around knee/1 -> Product1/2
  Product1/1 -> Sum2/2
  r(q) for HAM at knee/1 -> Sum2/1
  r(q) for HAM at hip/1 -> Sum1/3
  r(q) for GLU/1 -> Sum1/2
  r(q) for HFL/1 -> Sum1/1
  Sum1/1 -> tauHP [Nm]/1
  Demux1/7 -> Subsystem/1(F VAS), Product2/1  "VAS"
  Demux1/8 -> r(q) for BFSH/1  "BFSH"
  Demux1/9 -> Product3/1, Product4/1  "GAS"
  r(q) RGAS around knee/1 -> Product3/2
  Product2/1 -> Sum2/3
  r(q) for BFSH/1 -> Sum2/4
  Product3/1 -> Sum2/5
  Sum2/1 -> tauK [Nm]/1
  r(q) RGAS around ankle/1 -> Product4/2
  Demux1/10 -> Subsystem/3(F SOL), Product5/1  "SOL"
  r(q) RTA/1 -> Product6/2
  Demux1/11 -> Product6/1  "TA"
  Sum3/1 -> tauA [Nm]/1
  Sum/1 -> tauHR [Nm]/1
  Product6/1 -> Sum3/3
  Product4/1 -> Sum3/1
  Product5/1 -> Sum3/2
  r(q) for VAS/1 -> Subsystem/2(Moment Arm VAS), Product2/2
  r(q) RSOL/1 -> Subsystem/4(Moment Arm SOL), Product5/2
  Subsystem/1("Leg Torque ") -> Leg Torque/1
  Sum4/1 -> tauAR [Nm]/1
  r(q) for HAB1/1 -> Sum4/1
  Demux1/13 -> r(q) for HAD1/1  "EVE"
  Demux1/12 -> r(q) for HAB1/1  "INV"
  r(q) for HAD1/1 -> Sum4/2

== system nms3D_2021/Spinal Layer/Spinal Reflexes Control Left (Stance only)/L Stance Phase (coronal) ==
  note: Left Stance Phase Control
  note: M3: balance trunk old
  CompliantLegLat : Inport
  FmHAB : Inport  Port=2
  theta_tgt [rad] world : Inport  Port=3
  theta dtheta [rad rad/s] : Inport  Port=4
  BalanceTrunkLat old : Inport  Port=5
  Enable : EnablePort  StatesWhenEnabling=reset  ZeroCross=off
  Demux1 : Demux
  Demux7 : Demux  Outputs=2
  Divide{1..2,6..7,15} (5 alike) : Product
  Gain1 : Gain  Gain=-1
  Gain3 : Gain  Gain=-1
  Mux2 : Mux  Inputs=2
  Sum1 : Sum  Inputs=-+|  InputSameDT=on  SaturateOnIntegerOverflow=on  OutDataTypeStr=Inherit: Same as first input
  Sum5 : Sum  Inputs=|++  InputSameDT=on  SaturateOnIntegerOverflow=on  OutDataTypeStr=Inherit: Same as first input
  Sum6 : Sum  Inputs=|++  InputSameDT=on  SaturateOnIntegerOverflow=on  OutDataTypeStr=Inherit: Same as first input
  positive half3 : Saturate  UpperLimit=inf  LowerLimit=0  ZeroCross=off
  positive half4 : Saturate  UpperLimit=inf  LowerLimit=0  ZeroCross=off
  S_M1 [HAB] : Outport  OutputWhenDisabled=reset  InitialOutput=0  VectorParamsAs1DForOutWhenUnconnected=off
  S_M3 [HAB HAD] old : Outport  Port=2  OutputWhenDisabled=reset  InitialOutput=0  VectorParamsAs1DForOutWhenUnconnected=off
  wires:
  Divide7/1 -> S_M1 [HAB]/1  "HAB"
  FmHAB/1 -> Divide7/2
  CompliantLegLat/1 -> Divide7/1
  Gain1/1 -> Divide2/1
  theta dtheta [rad rad/s]/1 -> Demux7/1
  positive half4/1 -> Mux2/2
  positive half3/1 -> Mux2/1
  Sum5/1 -> positive half3/1  "HAB"
  Divide2/1 -> Sum5/1
  Gain3/1 -> Divide6/1
  Demux1/2 -> Divide6/2  "GainDTh_HAB"
  Demux1/4 -> Divide15/2  "GainDTh_HAD"
  Divide6/1 -> Sum5/2
  BalanceTrunkLat old/1 -> Demux1/1
  theta_tgt [rad] world/1 -> Sum1/1
  Divide1/1 -> Sum6/1
  Divide15/1 -> Sum6/2
  Demux7/1 -> Sum1/2  "theta"
  Demux1/1 -> Divide2/2  "GainTh_HAB"
  Sum1/1 -> Gain1/1, Divide1/1
  Mux2/1 -> S_M3 [HAB HAD] old/1
  Demux1/3 -> Divide1/2  "GainTh_HAD"
  Demux7/2 -> Gain3/1, Divide15/1  "dtheta"
  Sum6/1 -> positive half4/1  "HAD"

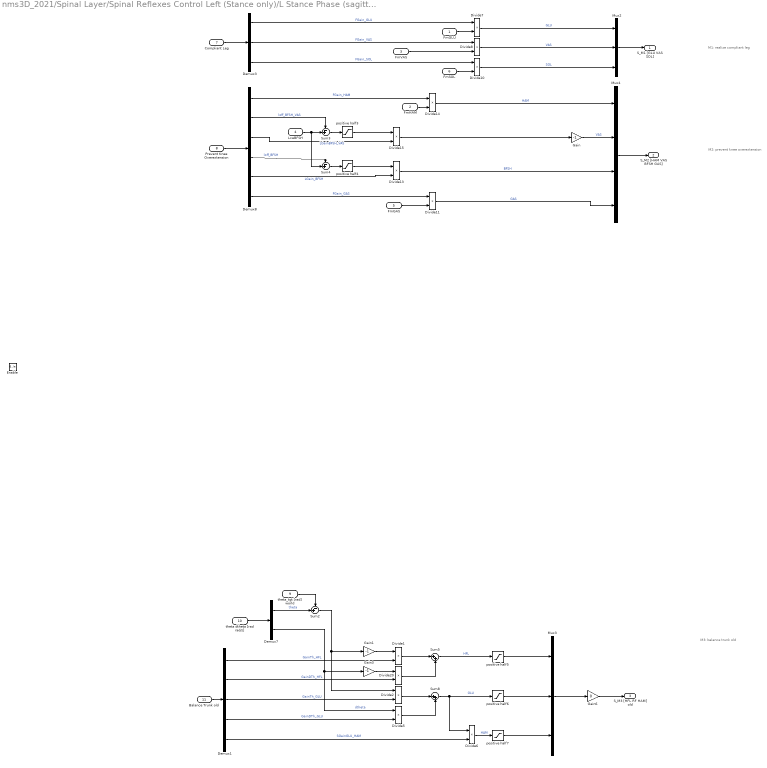
== system nms3D_2021/Spinal Layer/Spinal Reflexes Control Left (Stance only)/L Stance Phase (sagittal) ==
  note: M1: realize compliant leg
  note: M2: prevent knee overextension
  note: M3: balance trunk old
  FmGLU : Inport
  FmHAM : Inport  Port=2
  FmVAS : Inport  Port=3
  LceBFSH : Inport  Port=4
  FmGAS : Inport  Port=5
  FmSOL : Inport  Port=6
  Compliant Leg : Inport  Port=7
  Prevent Knee Overextension : Inport  Port=8
  theta_tgt [rad] world : Inport  Port=9
  theta dtheta [rad rad/s] : Inport  Port=10
  Balance Trunk old : Inport  Port=11
  Enable : EnablePort  StatesWhenEnabling=reset  ZeroCross=off
  Demux1 : Demux  Outputs=5
  Demux3 : Demux  Outputs=3
  Demux7 : Demux  Outputs=2
  Demux8 : Demux  Outputs=6
  Divide{1..2,5..8,10..11,13..15,20} (12 alike) : Product
  Gain : Gain  Gain=-1
  Gain1 : Gain  Gain=-1
  Gain3 : Gain  Gain=-1
  Gain6 : Gain  Gain=0
  Mux2 : Mux  Inputs=3
  Mux3 : Mux  Inputs=3
  Mux4 : Mux
  Sum2 : Sum  Inputs=-+|  InputSameDT=on  SaturateOnIntegerOverflow=on  OutDataTypeStr=Inherit: Same as first input
  Sum3 : Sum  Inputs=-+|  InputSameDT=on  SaturateOnIntegerOverflow=on  OutDataTypeStr=Inherit: Same as first input
  Sum4 : Sum  Inputs=-+|  InputSameDT=on  SaturateOnIntegerOverflow=on  OutDataTypeStr=Inherit: Same as first input
  Sum5 : Sum  Inputs=|++  InputSameDT=on  SaturateOnIntegerOverflow=on  OutDataTypeStr=Inherit: Same as first input
  Sum8 : Sum  Inputs=|++  InputSameDT=on  SaturateOnIntegerOverflow=on  OutDataTypeStr=Inherit: Same as first input
  positive half{3..7} (5 alike) : Saturate  UpperLimit=inf  LowerLimit=0  ZeroCross=off
  S_M1 [GLU VAS SOL] : Outport  OutputWhenDisabled=reset  InitialOutput=0  VectorParamsAs1DForOutWhenUnconnected=off
  S_M2 [HAM VAS BFSH GAS] : Outport  Port=2  OutputWhenDisabled=reset  InitialOutput=0  VectorParamsAs1DForOutWhenUnconnected=off
  S_M3 [HFL RF HAM] old : Outport  Port=3  OutputWhenDisabled=reset  InitialOutput=0  VectorParamsAs1DForOutWhenUnconnected=off
  wires:
  Demux3/2 -> Divide8/1  "FGain_VAS"
  Demux3/3 -> Divide10/1  "FGain_SOL"
  Divide10/1 -> Mux2/3  "SOL"
  Divide8/1 -> Mux2/2  "VAS"
  Demux3/1 -> Divide7/1  "FGain_GLU"
  Divide7/1 -> Mux2/1  "GLU"
  FmGLU/1 -> Divide7/2
  FmVAS/1 -> Divide8/2
  FmSOL/1 -> Divide10/2
  Prevent Knee Overextension/1 -> Demux8/1
  Sum3/1 -> positive half3/1
  Demux8/3 -> Divide15/2  "LGainBFSH_VAS"
  Demux8/5 -> Divide13/2  "LGain_BFSH"
  Demux8/6 -> Divide11/1  "FGain_GAS"
  positive half3/1 -> Divide15/1
  Demux8/2 -> Sum3/1  "loff_BFSH_VAS"
  Divide15/1 -> Gain/1
  Divide11/1 -> Mux4/4  "GAS"
  Demux8/1 -> Divide14/1  "FGain_HAM"
  Divide14/1 -> Mux4/1  "HAM"
  Gain/1 -> Mux4/2  "VAS"
  Sum4/1 -> positive half4/1
  positive half4/1 -> Divide13/1
  Demux8/4 -> Sum4/1  "loff_BFSH"
  FmHAM/1 -> Divide14/2
  LceBFSH/1 -> Sum3/2, Sum4/2
  FmGAS/1 -> Divide11/2
  Mux4/1 -> S_M2 [HAM VAS BFSH GAS]/1
  Compliant Leg/1 -> Demux3/1
  Mux2/1 -> S_M1 [GLU VAS SOL]/1
  Divide13/1 -> Mux4/3  "BFSH"
  Divide20/1 -> Sum5/2
  Divide5/1 -> Sum8/2
  theta dtheta [rad rad/s]/1 -> Demux7/1
  Demux1/4 -> Divide5/2  "GainDTh_GLU"
  Divide6/1 -> positive half7/1  "HAM"
  Demux7/1 -> Sum2/2  "theta"
  Demux7/2 -> Gain3/1, Divide5/1  "dtheta"
  Sum2/1 -> Gain1/1, Divide2/1
  Divide1/1 -> Sum5/1
  positive half6/1 -> Mux3/2
  Sum8/1 -> Divide6/1, positive half6/1  "GLU"
  Demux1/1 -> Divide1/2  "GainTh_HFL"
  Gain3/1 -> Divide20/1
  Sum5/1 -> positive half5/1  "HFL"
  Demux1/2 -> Divide20/2  "GainDTh_HFL"
  Mux3/1 -> Gain6/1
  Balance Trunk old/1 -> Demux1/1
  Demux1/3 -> Divide2/2  "GainTh_GLU"
  Demux1/5 -> Divide6/2  "SGainGLU_HAM"
  theta_tgt [rad] world/1 -> Sum2/1
  positive half7/1 -> Mux3/3
  positive half5/1 -> Mux3/1
  Gain1/1 -> Divide1/1
  Divide2/1 -> Sum8/1
  Gain6/1 -> S_M3 [HFL RF HAM] old/1

== system nms3D_2021/Spinal Layer/Spinal Reflexes Control Right (Stance only)/R Stance Phase (coronal) ==
  note: Left Stance Phase Control
  note: M3: balance trunk old
  CompliantLegLat : Inport
  FmHAB : Inport  Port=2
  theta_tgt [rad] world : Inport  Port=3
  theta dtheta [rad rad/s] : Inport  Port=4
  BalanceTrunkLat old : Inport  Port=5
  Enable : EnablePort  StatesWhenEnabling=reset  ZeroCross=off
  Demux1 : Demux
  Demux7 : Demux  Outputs=2
  Divide{1..2,6..7,15} (5 alike) : Product
  Gain1 : Gain  Gain=-1
  Gain3 : Gain  Gain=-1
  Mux2 : Mux  Inputs=2
  Sum1 : Sum  Inputs=-+|  InputSameDT=on  SaturateOnIntegerOverflow=on  OutDataTypeStr=Inherit: Same as first input
  Sum5 : Sum  Inputs=|++  InputSameDT=on  SaturateOnIntegerOverflow=on  OutDataTypeStr=Inherit: Same as first input
  Sum6 : Sum  Inputs=|++  InputSameDT=on  SaturateOnIntegerOverflow=on  OutDataTypeStr=Inherit: Same as first input
  positive half3 : Saturate  UpperLimit=inf  LowerLimit=0  ZeroCross=off
  positive half4 : Saturate  UpperLimit=inf  LowerLimit=0  ZeroCross=off
  S_M1 [HAB] : Outport  OutputWhenDisabled=reset  InitialOutput=0  VectorParamsAs1DForOutWhenUnconnected=off
  S_M3 [HAB HAD] old : Outport  Port=2  OutputWhenDisabled=reset  InitialOutput=0  VectorParamsAs1DForOutWhenUnconnected=off
  wires:
  Divide7/1 -> S_M1 [HAB]/1  "HAB"
  FmHAB/1 -> Divide7/2
  CompliantLegLat/1 -> Divide7/1
  Gain1/1 -> Divide2/1
  theta dtheta [rad rad/s]/1 -> Demux7/1
  positive half4/1 -> Mux2/2
  positive half3/1 -> Mux2/1
  Sum5/1 -> positive half3/1  "HAB"
  Divide2/1 -> Sum5/1
  Gain3/1 -> Divide6/1
  Demux1/2 -> Divide6/2  "GainDTh_HAB"
  Demux1/4 -> Divide15/2  "GainDTh_HAD"
  Divide6/1 -> Sum5/2
  BalanceTrunkLat old/1 -> Demux1/1
  theta_tgt [rad] world/1 -> Sum1/1
  Divide1/1 -> Sum6/1
  Divide15/1 -> Sum6/2
  Demux7/1 -> Sum1/2  "theta"
  Demux1/1 -> Divide2/2  "GainTh_HAB"
  Sum1/1 -> Gain1/1, Divide1/1
  Mux2/1 -> S_M3 [HAB HAD] old/1
  Demux1/3 -> Divide1/2  "GainTh_HAD"
  Demux7/2 -> Gain3/1, Divide15/1  "dtheta"
  Sum6/1 -> positive half4/1  "HAD"

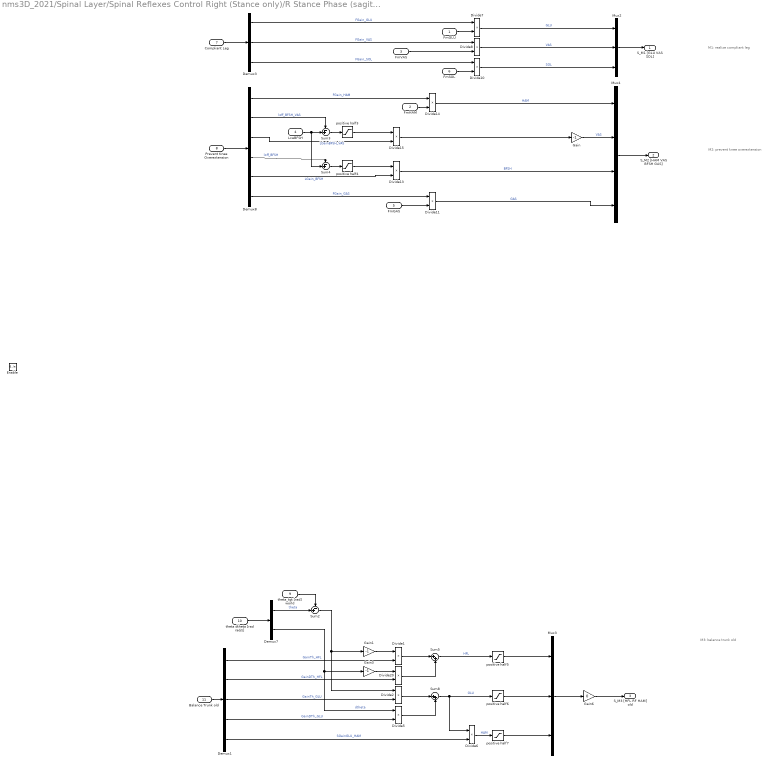
== system nms3D_2021/Spinal Layer/Spinal Reflexes Control Right (Stance only)/R Stance Phase (sagittal) ==
  note: M1: realize compliant leg
  note: M2: prevent knee overextension
  note: M3: balance trunk old
  FmGLU : Inport
  FmHAM : Inport  Port=2
  FmVAS : Inport  Port=3
  LceBFSH : Inport  Port=4
  FmGAS : Inport  Port=5
  FmSOL : Inport  Port=6
  Compliant Leg : Inport  Port=7
  Prevent Knee Overextension : Inport  Port=8
  theta_tgt [rad] world : Inport  Port=9
  theta dtheta [rad rad/s] : Inport  Port=10
  Balance Trunk old : Inport  Port=11
  Enable : EnablePort  StatesWhenEnabling=reset  ZeroCross=off
  Demux1 : Demux  Outputs=5
  Demux3 : Demux  Outputs=3
  Demux7 : Demux  Outputs=2
  Demux8 : Demux  Outputs=6
  Divide{1..2,5..8,10..11,13..15,20} (12 alike) : Product
  Gain : Gain  Gain=-1
  Gain1 : Gain  Gain=-1
  Gain3 : Gain  Gain=-1
  Gain6 : Gain  Gain=0
  Mux2 : Mux  Inputs=3
  Mux3 : Mux  Inputs=3
  Mux4 : Mux
  Sum2 : Sum  Inputs=-+|  InputSameDT=on  SaturateOnIntegerOverflow=on  OutDataTypeStr=Inherit: Same as first input
  Sum3 : Sum  Inputs=-+|  InputSameDT=on  SaturateOnIntegerOverflow=on  OutDataTypeStr=Inherit: Same as first input
  Sum4 : Sum  Inputs=-+|  InputSameDT=on  SaturateOnIntegerOverflow=on  OutDataTypeStr=Inherit: Same as first input
  Sum5 : Sum  Inputs=|++  InputSameDT=on  SaturateOnIntegerOverflow=on  OutDataTypeStr=Inherit: Same as first input
  Sum8 : Sum  Inputs=|++  InputSameDT=on  SaturateOnIntegerOverflow=on  OutDataTypeStr=Inherit: Same as first input
  positive half{3..7} (5 alike) : Saturate  UpperLimit=inf  LowerLimit=0  ZeroCross=off
  S_M1 [GLU VAS SOL] : Outport  OutputWhenDisabled=reset  InitialOutput=0  VectorParamsAs1DForOutWhenUnconnected=off
  S_M2 [HAM VAS BFSH GAS] : Outport  Port=2  OutputWhenDisabled=reset  InitialOutput=0  VectorParamsAs1DForOutWhenUnconnected=off
  S_M3 [HFL RF HAM] old : Outport  Port=3  OutputWhenDisabled=reset  InitialOutput=0  VectorParamsAs1DForOutWhenUnconnected=off
  wires:
  Demux3/2 -> Divide8/1  "FGain_VAS"
  Demux3/3 -> Divide10/1  "FGain_SOL"
  Divide10/1 -> Mux2/3  "SOL"
  Divide8/1 -> Mux2/2  "VAS"
  Demux3/1 -> Divide7/1  "FGain_GLU"
  Divide7/1 -> Mux2/1  "GLU"
  FmGLU/1 -> Divide7/2
  FmVAS/1 -> Divide8/2
  FmSOL/1 -> Divide10/2
  Prevent Knee Overextension/1 -> Demux8/1
  Sum3/1 -> positive half3/1
  Demux8/3 -> Divide15/2  "LGainBFSH_VAS"
  Demux8/5 -> Divide13/2  "LGain_BFSH"
  Demux8/6 -> Divide11/1  "FGain_GAS"
  positive half3/1 -> Divide15/1
  Demux8/2 -> Sum3/1  "loff_BFSH_VAS"
  Divide15/1 -> Gain/1
  Divide11/1 -> Mux4/4  "GAS"
  Demux8/1 -> Divide14/1  "FGain_HAM"
  Divide14/1 -> Mux4/1  "HAM"
  Gain/1 -> Mux4/2  "VAS"
  Sum4/1 -> positive half4/1
  positive half4/1 -> Divide13/1
  Demux8/4 -> Sum4/1  "loff_BFSH"
  FmHAM/1 -> Divide14/2
  LceBFSH/1 -> Sum3/2, Sum4/2
  FmGAS/1 -> Divide11/2
  Mux4/1 -> S_M2 [HAM VAS BFSH GAS]/1
  Compliant Leg/1 -> Demux3/1
  Mux2/1 -> S_M1 [GLU VAS SOL]/1
  Divide13/1 -> Mux4/3  "BFSH"
  Divide20/1 -> Sum5/2
  Divide5/1 -> Sum8/2
  theta dtheta [rad rad/s]/1 -> Demux7/1
  Demux1/4 -> Divide5/2  "GainDTh_GLU"
  Divide6/1 -> positive half7/1  "HAM"
  Demux7/1 -> Sum2/2  "theta"
  Demux7/2 -> Gain3/1, Divide5/1  "dtheta"
  Sum2/1 -> Gain1/1, Divide2/1
  Divide1/1 -> Sum5/1
  positive half6/1 -> Mux3/2
  Sum8/1 -> Divide6/1, positive half6/1  "GLU"
  Demux1/1 -> Divide1/2  "GainTh_HFL"
  Gain3/1 -> Divide20/1
  Sum5/1 -> positive half5/1  "HFL"
  Demux1/2 -> Divide20/2  "GainDTh_HFL"
  Mux3/1 -> Gain6/1
  Balance Trunk old/1 -> Demux1/1
  Demux1/3 -> Divide2/2  "GainTh_GLU"
  Demux1/5 -> Divide6/2  "SGainGLU_HAM"
  theta_tgt [rad] world/1 -> Sum2/1
  positive half7/1 -> Mux3/3
  positive half5/1 -> Mux3/1
  Gain1/1 -> Divide1/1
  Divide2/1 -> Sum8/1
  Gain6/1 -> S_M3 [HFL RF HAM] old/1

== system nms3D_2021/Spinal Layer/Stretch Reflex/Stretch Reflex Left ==
  lambda : Inport
  l_ce : Inport  Port=2
  v_ce : Inport  Port=3
  lambda_dot : Inport  Port=4
  Add2 : Sum  Inputs=-+
  Add3 : Sum  Inputs=-+
  Add7 : Sum
  Gain10 : Gain  Gain=0.03
  Gain9 : Gain  Gain=mParams.muscles.K
  STIM : Outport  VectorParamsAs1DForOutWhenUnconnected=off
  wires:
  lambda/1 -> Add2/1
  Add7/1 -> STIM/1
  Gain9/1 -> Add7/1
  Gain10/1 -> Add7/2
  Add3/1 -> Gain10/1
  Add2/1 -> Gain9/1
  v_ce/1 -> Add3/2
  l_ce/1 -> Add2/2
  lambda_dot/1 -> Add3/1

== system nms3D_2021/Spinal Layer/Stretch Reflex/Stretch Reflex Right ==
  lambda : Inport
  l_ce : Inport  Port=2
  v_ce : Inport  Port=3
  lambda_dot : Inport  Port=4
  Add2 : Sum  Inputs=-+
  Add3 : Sum  Inputs=-+
  Add7 : Sum
  Gain1 : Gain  Commented=on  Gain=[ 0.03 0.03 0.03 0.03 0.03 0.03 0.03 0.03 0.1 0.1 0.1]
  Gain10 : Gain  Gain=0.03
  Gain9 : Gain  Gain=mParams.muscles.K
  STIM : Outport  VectorParamsAs1DForOutWhenUnconnected=off
  wires:
  lambda/1 -> Add2/1
  Add7/1 -> STIM/1
  Gain9/1 -> Add7/1
  Gain10/1 -> Add7/2
  Add3/1 -> Gain10/1
  Add2/1 -> Gain9/1
  v_ce/1 -> Add3/2
  l_ce/1 -> Add2/2
  lambda_dot/1 -> Add3/1

== system nms3D_2021/Supraspinal Level/Subsystem/Compute positives forces that generate desired torque profiles1 ==
  note: Desired Forces: Desired Forces are computed by an iterative approach. The pseudoinverse-method is used to compute forces that generate the desired force profiles. This forces, however, can potentially be negative unlike real muscle forces. Therefore, torques that these negative forces would produce are computed. The resulting torques are again transformed into forces that have a smaller negative component now. This procedure is repeated 6 times.
  Left/Right : Inport
  Stance Left : Inport  Port=2
  Swing Left : Inport  Port=3
  Swing Right : Inport  Port=4
  Stance Right : Inport  Port=5
  Left : Subsystem
  Mux1 : Mux  Inputs=2
  Right : Subsystem
  Switch6 : Switch  Criteria=u2 > Threshold
  Switch7 : Switch  Criteria=u2 > Threshold
  Desired Force : Outport
  wires:
  ? -> ?
  [Llegq] -> Left/2(Angles)
  [Rlegq] -> Right/2(Angles)
  Switch6/1 -> Left/1(Desired Torques)
  Switch7/1 -> Right/1(Desired Torques)
  Swing Right/1 -> Switch7/1
  Swing Left/1 -> Switch6/3
  Stance Left/1 -> Switch6/1
  Stance Right/1 -> Switch7/3
  Mux1/1 -> Desired Force/1
  Left/Right/1 -> Switch6/2, Switch7/2
  Left/1(Forces) -> Mux1/1
  Right/1(Forces) -> Mux1/2

== system nms3D_2021/Supraspinal Level/Subsystem/Inversion of Muscle Model ==
  note: Inversion of Muscle Model: This block implements the inversion of the Hill-type muscle model.
  Desired Forces : Inport
  Divide1 : Product  Inputs=*/
  Divide11 : Product  Inputs=*/
  Fmax1 : Gain  Gain=1./mParams.muscles.FmaxVec  SaturateOnIntegerOverflow=on  OutDataTypeStr=Inherit: Same as input  ParamDataTypeStr=Inherit: Same as input
  Fmax4 : Gain  Gain=1./mParams.muscles.FmaxVec  SaturateOnIntegerOverflow=on  OutDataTypeStr=Inherit: Same as input  ParamDataTypeStr=Inherit: Same as input
  Multiply2 : Product
  Multiply6 : Product
  Saturation{1..3,5} (4 alike) : Saturate  UpperLimit=inf  LowerLimit=0.00005  ZeroCross=off
  Selector : Selector  InputPortWidth=26  IndexOptions=Index vector (dialog)  Indices=[1:13]  OutputSizes=1
  Selector1 : Selector  InputPortWidth=26  IndexOptions=Index vector (dialog)  Indices=[14:26]  OutputSizes=1
  Desired Activation Left : Outport
  Desired Activation Right : Outport  Port=2
  wires:
  Saturation1/1 -> Multiply6/1
  Multiply6/1 -> Divide11/2
  [fl_R] -> Saturation2/1
  [fl_L] -> Saturation5/1
  Fmax4/1 -> Divide11/1
  Saturation3/1 -> Multiply2/1
  [fv_R] -> Saturation1/1
  Saturation5/1 -> Multiply2/2
  [fv_L] -> Saturation3/1
  Multiply2/1 -> Divide1/2
  Saturation2/1 -> Multiply6/2
  Fmax1/1 -> Divide1/1
  Divide1/1 -> Desired Activation Left/1
  Divide11/1 -> Desired Activation Right/1
  Selector/1 -> Fmax1/1
  Selector1/1 -> Fmax4/1
  Desired Forces/1 -> Selector1/1, Selector/1

== system nms3D_2021/Supraspinal Level/Subsystem/Stance Leg Control ==
  note: Wrench to be generated by Left/Right Stance Leg
  Left/Right : Inport
  Balance Control Equation [Ankle Strategy] : Subsystem
  Coordiante Transform Interaction Wrenches : Subsystem  Commented=on
  PD-Controller For Saggital Trunk Balance : Subsystem
  Stance Leg : Subsystem
  long delay 1 : eeGeneralControl/Low-Pass Filter (Discrete or Continuous)  K=1  T=mParams.control.delays.long  B=inf  A=-inf  init_option=Inherited from block input  x0=0  Ts=-1
  long delay 2 : eeGeneralControl/Low-Pass Filter (Discrete or Continuous)  K=1  T=mParams.control.delays.long  B=inf  A=-inf  init_option=Inherited from block input  x0=0  Ts=-1
  Push Off Left : Outport
  Push Off Right : Outport  Port=2
  wires:
  Left/Right/1 -> Stance Leg/1(left/right), Coordiante Transform Interaction Wrenches/3(Left/Right)
  Stance Leg/1(Stance Torques Left) -> long delay 1/1
  Stance Leg/2(Stance Torques Right) -> long delay 2/1
  long delay 1/1 -> Push Off Left/1
  long delay 2/1 -> Push Off Right/1
  Balance Control Equation [Ankle Strategy]/1(Desired Acceleration (CoM)) -> Stance Leg/2(Balance Control [Ankle Strategy])
  PD-Controller For Saggital Trunk Balance/1(PD Input) -> Stance Leg/3(PD Input)

== system nms3D_2021/Supraspinal Level/Subsystem/Stretch Reflex Inversion ==
  note: Inversion of Stretch: This block implements the inversion of the tonic stretch reflex.
  Desired Activation Left : Inport
  Desired Activation Right : Inport  Port=2
  Gain1 : Gain  Gain=-1/mParams.muscles.K
  Gain12 : Gain  Gain=-1/mParams.muscles.K
  Sum14 : Sum  Inputs=|++
  Sum2 : Sum  Inputs=|++
  Descending Command Left : Outport
  Descending Command Right : Outport  Port=2
  wires:
  Desired Activation Right/1 -> Gain12/1
  Sum14/1 -> Descending Command Right/1
  Desired Activation Left/1 -> Gain1/1
  Sum2/1 -> Descending Command Left/1
  [RLceVec] -> Sum14/2
  Gain12/1 -> Sum14/1
  Gain1/1 -> Sum2/1
  [LLceVec] -> Sum2/2
